simulink model "PGS_STD_SINV_MODEL_Rectifier_2022b"  (R2022b)
settings: Solver=VariableStepAuto  StartTime=0.0  StopTime=4.0  RelTol=1e-3
PostLoadFcn:
  | gmp_model_file=get_param(bdroot,'FileName'); if isempty(gmp_model_file), error('GMP:SINV:ModelPath', 'The SINV model must be saved before SDPE initialization.'); end; gmp_model_dir=fileparts(gmp_model_file); run(fullfile(gmp_model_dir,'..','..','sdpe_general','sdpe_pgs_sinv_rc_common_settings_matlab_init.m')); run(fullfile(gmp_model_dir,'sdpe_mgr','sdpe_pgs_sinv_rc_simulate_settings_matlab_init.m')); addpath(fullfile(gmp_model_dir,'..','..','..','..','..','tools','gmp_sil','udp_helper_v2','mdl_asio_helper','bin','x64','Debug')); clear gmp_model_file gmp_model_dir;
InitFcn:
  | gmp_model_file=get_param(bdroot,'FileName'); if isempty(gmp_model_file), error('GMP:SINV:ModelPath', 'The SINV model must be saved before SDPE initialization.'); end; gmp_model_dir=fileparts(gmp_model_file); run(fullfile(gmp_model_dir,'..','..','sdpe_general','sdpe_pgs_sinv_rc_common_settings_matlab_init.m')); run(fullfile(gmp_model_dir,'sdpe_mgr','sdpe_pgs_sinv_rc_simulate_settings_matlab_init.m')); addpath(fullfile(gmp_model_dir,'..','..','..','..','..','tools','gmp_sil','udp_helper_v2','mdl_asio_helper','bin','x64','Debug')); clear gmp_model_file gmp_model_dir;
undefined symbols (not defined in the file or in its folder): CTRL_AC_CURRENT_BIAS, CTRL_AC_CURRENT_SENSITIVITY, CTRL_AC_INDUCTANCE, CTRL_AC_RESISTANCE, CTRL_AC_VOLTAGE_BIAS, CTRL_AC_VOLTAGE_SENSITIVITY, CTRL_ADC_RESOLUTION, CTRL_ADC_VOLTAGE_REF, CTRL_DC_VOLTAGE_BIAS, CTRL_DC_VOLTAGE_SENSITIVITY, CTRL_GRID_FREQUENCY, CTRL_GRID_VOLTAGE_RMS, CTRL_PWM_CMP_MAX, CTRL_PWM_DEADBAND_CMP, powergui, SINV_DC_CAPACITANCE_F, SINV_FILTER_CAP_ESR_OHM, SINV_FILTER_CAPACITANCE_F, SINV_MODEL_DIODE_RON, SINV_MODEL_DIODE_VF, SINV_MODEL_MOSFET_RON, SINV_PWM_FREQUENCY_HZ, SINV_RECTIFIER_RLOAD_OHM, sps_lib
libraries: spsSeriesRLCBranchLib x9, spsVoltageMeasurementLib x6, spsSecondOrderFilterLib x5, gmp_peripheral_utilities x2, gmp_sil_core_pack x1, spsControlledVoltageSourceLib x1, spsCurrentMeasurementLib x1
(part 2 of 2)

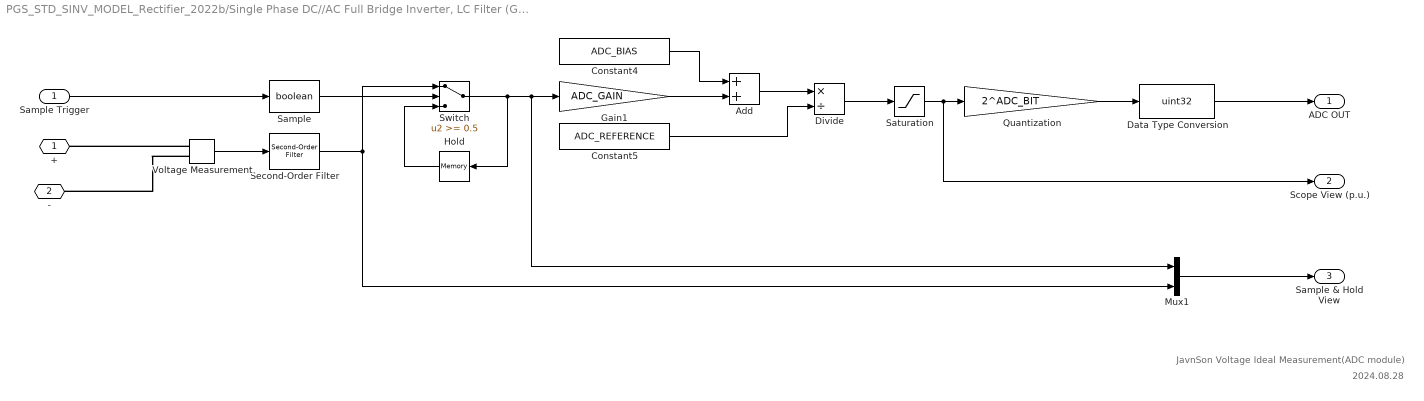
== system PGS_STD_SINV_MODEL_Rectifier_2022b/Single Phase DC//AC Full Bridge Inverter, LC Filter (GMP STD MDL)/DC bus Voltage Measurement Module ==
  note: JavnSon Voltage Ideal Measurement(ADC module)
  note: 2024.08.28
  Sample Trigger : Inport
  Add : Sum
  Constant4 : Constant  Value=ADC_BIAS
  Constant5 : Constant  Value=ADC_REFERENCE
  Data Type Conversion : DataTypeConversion  OutDataTypeStr=uint32  ConvertRealWorld=Stored Integer (SI)  SaturateOnIntegerOverflow=off  RndMeth=Floor
  Divide : Product  Inputs=*/
  Gain1 : Gain  Gain=ADC_GAIN
  Hold : Memory  InitialCondition=ADC_INIT  LinearizeAsDelay=on
  Mux1 : Mux  Inputs=2
  Quantization : Gain  Gain=2^ADC_BIT
  Sample : DataTypeConversion  OutDataTypeStr=boolean  SaturateOnIntegerOverflow=off  RndMeth=Floor
  Saturation : Saturate  UpperLimit=1  LowerLimit=0
  Second-Order Filter : spsSecondOrderFilterLib/Second-Order Filter  FilterType=Lowpass  Fo=cut_frequency  Zeta=0.707  Ts=0  Initialize=off  Vac_Init="[0,  0,  60]"  Vdc_Init=0  PlotResponse=off  FreqRange=[0, 500, 1]
  Switch : Switch  Threshold=0.5
  Voltage Measurement : spsVoltageMeasurementLib/Voltage Measurement  PhasorSimulation=off  OutputType=Complex  PSBequivalent=0
  + : PMIOPort  Side=Left
  - : PMIOPort  Port=2  Side=Left
  ADC OUT : Outport
  Scope View (p.u.) : Outport  Port=2
  Sample & Hold View : Outport  Port=3
  wires:
  Second-Order Filter/1 -> Mux1/2, Switch/1
  Hold/1 -> Switch/3
  Switch/1 -> Hold/1, Mux1/1, Gain1/1
  Divide/1 -> Saturation/1
  Voltage Measurement/1 -> Second-Order Filter/1
  Saturation/1 -> Scope View (p.u.)/1, Quantization/1
  Constant4/1 -> Add/1
  Gain1/1 -> Add/2
  Sample Trigger/1 -> Sample/1
  Data Type Conversion/1 -> ADC OUT/1
  Mux1/1 -> Sample & Hold View/1
  Quantization/1 -> Data Type Conversion/1
  Constant5/1 -> Divide/2
  Add/1 -> Divide/1
  Sample/1 -> Switch/2
  connections:
  Voltage Measurement/LConn1 -- +/RConn1
  Voltage Measurement/LConn2 -- -/RConn1

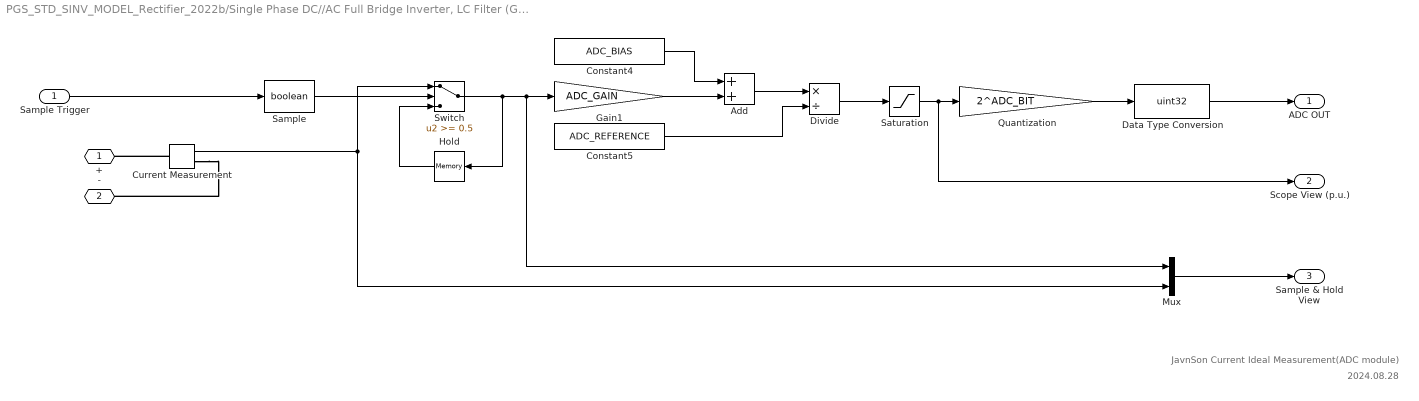
== system PGS_STD_SINV_MODEL_Rectifier_2022b/Single Phase DC//AC Full Bridge Inverter, LC Filter (GMP STD MDL)/Ideal Inductor Current Measurement Module（ADC - Current） ==
  note: JavnSon Current Ideal Measurement(ADC module)
  note: 2024.08.28
  Sample Trigger : Inport
  Add : Sum
  Constant4 : Constant  Value=ADC_BIAS
  Constant5 : Constant  Value=ADC_REFERENCE
  Current Measurement : spsCurrentMeasurementLib/Current Measurement  PhasorSimulation=off  OutputType=Complex  PSBequivalent=0
  Data Type Conversion : DataTypeConversion  OutDataTypeStr=uint32  ConvertRealWorld=Stored Integer (SI)  SaturateOnIntegerOverflow=off  RndMeth=Floor
  Divide : Product  Inputs=*/
  Gain1 : Gain  Gain=ADC_GAIN
  Hold : Memory  InitialCondition=ADC_INIT  LinearizeAsDelay=on
  Mux : Mux  Inputs=2
  Quantization : Gain  Gain=2^ADC_BIT
  Sample : DataTypeConversion  OutDataTypeStr=boolean  SaturateOnIntegerOverflow=off  RndMeth=Floor
  Saturation : Saturate  UpperLimit=1  LowerLimit=0
  Switch : Switch  Threshold=0.5
  + : PMIOPort  Side=Left
  - : PMIOPort  Port=2  Side=Right
  ADC OUT : Outport
  Scope View (p.u.) : Outport  Port=2
  Sample & Hold View : Outport  Port=3
  wires:
  Constant5/1 -> Divide/2
  Quantization/1 -> Data Type Conversion/1
  Sample/1 -> Switch/2
  Add/1 -> Divide/1
  Sample Trigger/1 -> Sample/1
  Data Type Conversion/1 -> ADC OUT/1
  Hold/1 -> Switch/3
  Current Measurement/1 -> Mux/2, Switch/1
  Constant4/1 -> Add/1
  Switch/1 -> Hold/1, Mux/1, Gain1/1
  Gain1/1 -> Add/2
  Saturation/1 -> Scope View (p.u.)/1, Quantization/1
  Divide/1 -> Saturation/1
  Mux/1 -> Sample & Hold View/1
  connections:
  Current Measurement/LConn1 -- +/RConn1
  Current Measurement/RConn1 -- -/RConn1

== system PGS_STD_SINV_MODEL_Rectifier_2022b/powergui/EquivalentModel1 ==
  Gates : Subsystem
  Sources : Subsystem
  State-Space : S-Function  FunctionName=sfun_spssw_discc  Parameters=S.Ts,S.A, S.B, S.C, S.D, S.x0, S.EnableUseOfTLC,S.SwitchResistance ,S.SwitchType, S.SwitchGateInitialValue, S.OutputsToResetToZero, S.TBEON,S.SaveMatrices,S.BufferSize  SFunctionDeploymentMode=off  EnableBusSupport=off
  Status : Subsystem
  Yout : Subsystem
  wires:
  Gates/1(gates) -> State-Space/2
  Sources/1(u) -> State-Space/1
  State-Space/2 -> Status/1(status)
  State-Space/1 -> Yout/1(v,i)

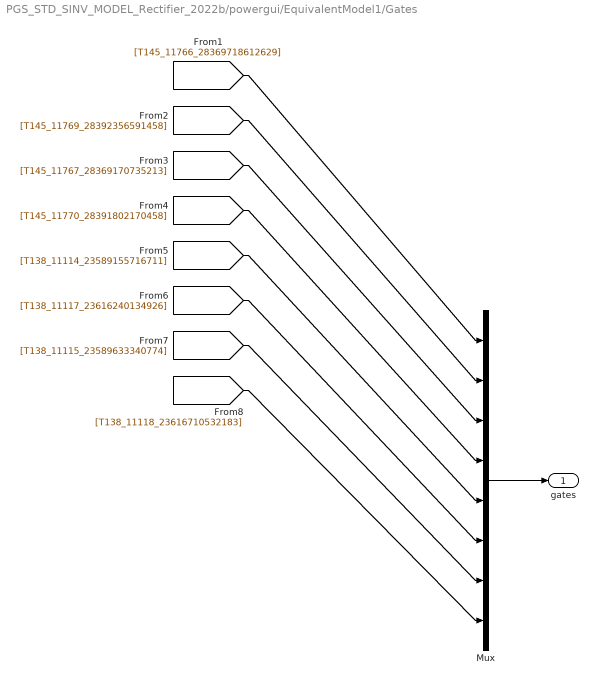
== system PGS_STD_SINV_MODEL_Rectifier_2022b/powergui/EquivalentModel1/Gates ==
  Mux : Mux  Inputs=[1 1 1 1 1 1 1 1]
  gates : Outport  VectorParamsAs1DForOutWhenUnconnected=off
  wires:
  Mux/1 -> gates/1
  [T145_11766_28369718612629] -> Mux/1
  [T145_11769_28392356591458] -> Mux/2
  [T145_11767_28369170735213] -> Mux/3
  [T145_11770_28391802170458] -> Mux/4
  [T138_11114_23589155716711] -> Mux/5
  [T138_11117_23616240134926] -> Mux/6
  [T138_11115_23589633340774] -> Mux/7
  [T138_11118_23616710532183] -> Mux/8

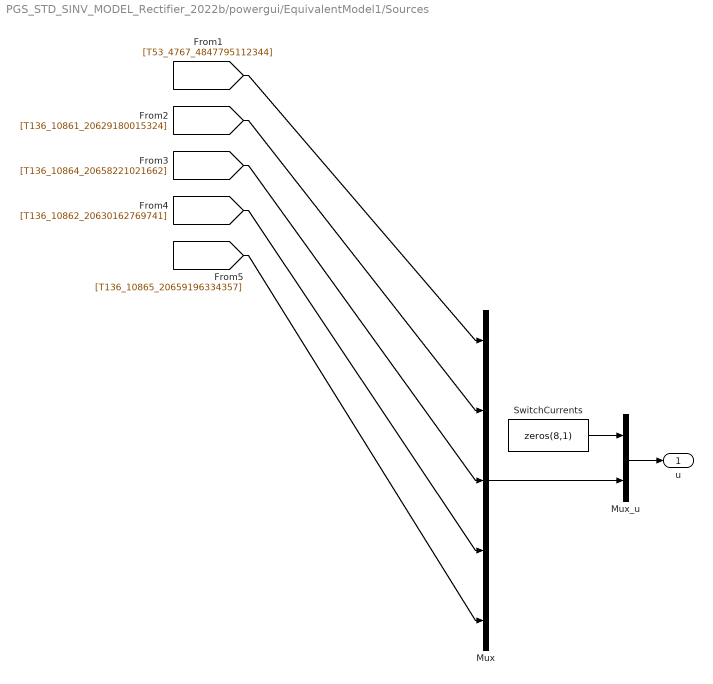
== system PGS_STD_SINV_MODEL_Rectifier_2022b/powergui/EquivalentModel1/Sources ==
  Mux : Mux  Inputs=[1 1 1 1 1]
  Mux_u : Mux  Inputs=[8 5]
  SwitchCurrents : Constant  Value=zeros(8,1)
  u : Outport  VectorParamsAs1DForOutWhenUnconnected=off
  wires:
  Mux_u/1 -> u/1
  SwitchCurrents/1 -> Mux_u/1
  Mux/1 -> Mux_u/2
  [T53_4767_4847795112344] -> Mux/1
  [T136_10861_20629180015324] -> Mux/2
  [T136_10864_20658221021662] -> Mux/3
  [T136_10862_20630162769741] -> Mux/4
  [T136_10865_20659196334357] -> Mux/5

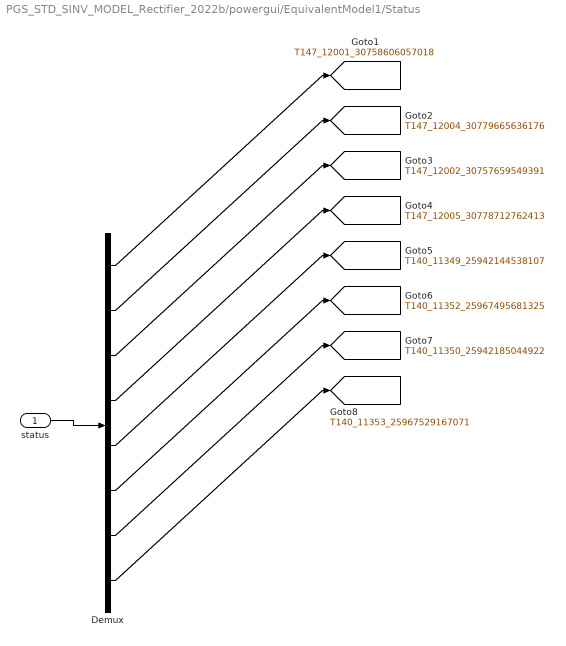
== system PGS_STD_SINV_MODEL_Rectifier_2022b/powergui/EquivalentModel1/Status ==
  status : Inport
  Demux : Demux  Outputs=[1 1 1 1 1 1 1 1]
  tag scope: T140_11349_25942144538107=global, T140_11350_25942185044922=global, T140_11352_25967495681325=global, T140_11353_25967529167071=global, T147_12001_30758606057018=global, T147_12002_30757659549391=global, T147_12004_30779665636176=global, T147_12005_30778712762413=global
  wires:
  status/1 -> Demux/1
  Demux/1 -> [T147_12001_30758606057018]
  Demux/2 -> [T147_12004_30779665636176]
  Demux/3 -> [T147_12002_30757659549391]
  Demux/4 -> [T147_12005_30778712762413]
  Demux/5 -> [T140_11349_25942144538107]
  Demux/6 -> [T140_11352_25967495681325]
  Demux/7 -> [T140_11350_25942185044922]
  Demux/8 -> [T140_11353_25967529167071]

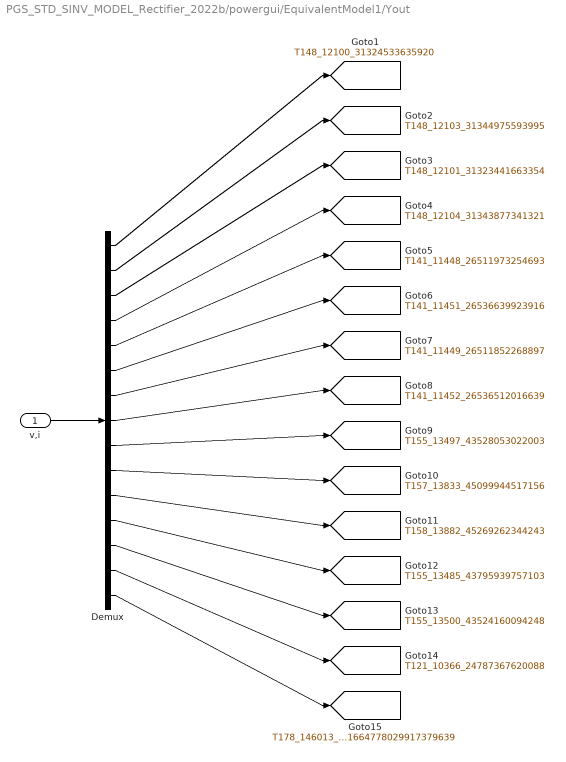
== system PGS_STD_SINV_MODEL_Rectifier_2022b/powergui/EquivalentModel1/Yout ==
  v,i : Inport
  Demux : Demux  Outputs=[1 1 1 1 1 1 1 1 1 1 1 1 1 1 1]
  tag scope: T121_10366_24787367620088=global, T141_11448_26511973254693=global, T141_11449_26511852268897=global, T141_11451_26536639923916=global, T141_11452_26536512016639=global, T148_12100_31324533635920=global, T148_12101_31323441663354=global, T148_12103_31344975593995=global, T148_12104_31343877341321=global, T155_13485_43795939757103=global, T155_13497_43528053022003=global, T155_13500_43524160094248=global, T157_13833_45099944517156=global, T158_13882_45269262344243=global, T178_146013_1664778029917379639=global
  wires:
  v,i/1 -> Demux/1
  Demux/1 -> [T148_12100_31324533635920]
  Demux/2 -> [T148_12103_31344975593995]
  Demux/3 -> [T148_12101_31323441663354]
  Demux/4 -> [T148_12104_31343877341321]
  Demux/5 -> [T141_11448_26511973254693]
  Demux/6 -> [T141_11451_26536639923916]
  Demux/7 -> [T141_11449_26511852268897]
  Demux/8 -> [T141_11452_26536512016639]
  Demux/9 -> [T155_13497_43528053022003]
  Demux/10 -> [T157_13833_45099944517156]
  Demux/11 -> [T158_13882_45269262344243]
  Demux/12 -> [T155_13485_43795939757103]
  Demux/13 -> [T155_13500_43524160094248]
  Demux/14 -> [T121_10366_24787367620088]
  Demux/15 -> [T178_146013_1664778029917379639]
